simulink model "tractioncontrol_rmse22"  (R2022a)
settings: Solver=VariableStepAuto  StartTime=0.0  StopTime=48  RelTol=1e-3
values from neighbouring files (symbols this model uses):
  A = 1.08    [test_script.m]
  c = 0.008    [test_script.m]
  Cd = 1.02    [test_script.m]
  g = 9.81    [test_script.m]
  gr = 47/13    (= 3.61538461538)    [test_script.m]
  h_cg = .259    (= 0.259)    [test_script.m]
  h_d = h_cg    (= 0.259)    [test_script.m]
  J = 0.27    [test_script.m]
  m = 297    [test_script.m]
  r = 0.5588    [test_script.m]
  rho = 1.162    [test_script.m]
  wb = 1.53    [test_script.m]
undefined symbols (not defined in the file or in its folder): efficiency, front_wb, simulation_results, uff
libraries: slpidlib x2
settings Model: Creator=sahil  LastModifiedBy=sahil

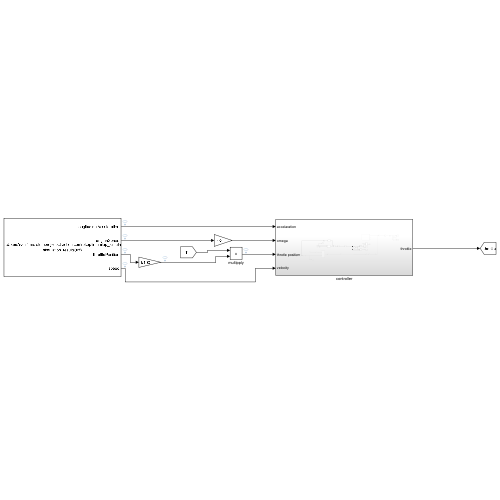
[thumbnail: Simulink's stored preview of the top-level diagram]
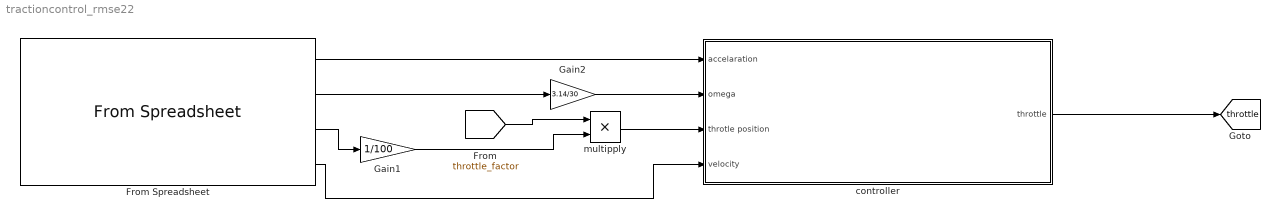
== system tractioncontrol_rmse22 ==
  From Spreadsheet : FromSpreadsheet  FileName=C:\Users\sahil\rms stuff\projects\traction control\optimumlap_simulations\simulation_results(uff).csv  SheetName=simulation_results(uff)
  Gain1 : Gain  Gain=1/100
  Gain2 : Gain  Gain=3.14/30
  controller : Subsystem
  multipply : Product  Inputs=**
  tag scope: throttle=global
  wires:
  From Spreadsheet/1 -> controller/1(accelaration)
  From Spreadsheet/3 -> Gain1/1
  controller/1(throttle) -> [throttle]
  From Spreadsheet/2 -> Gain2/1
  From Spreadsheet/4 -> controller/4(velocity)
  Gain2/1 -> controller/2(omega)
  [throttle_factor] -> multipply/1
  Gain1/1 -> multipply/2
  multipply/1 -> controller/3(throtle position)

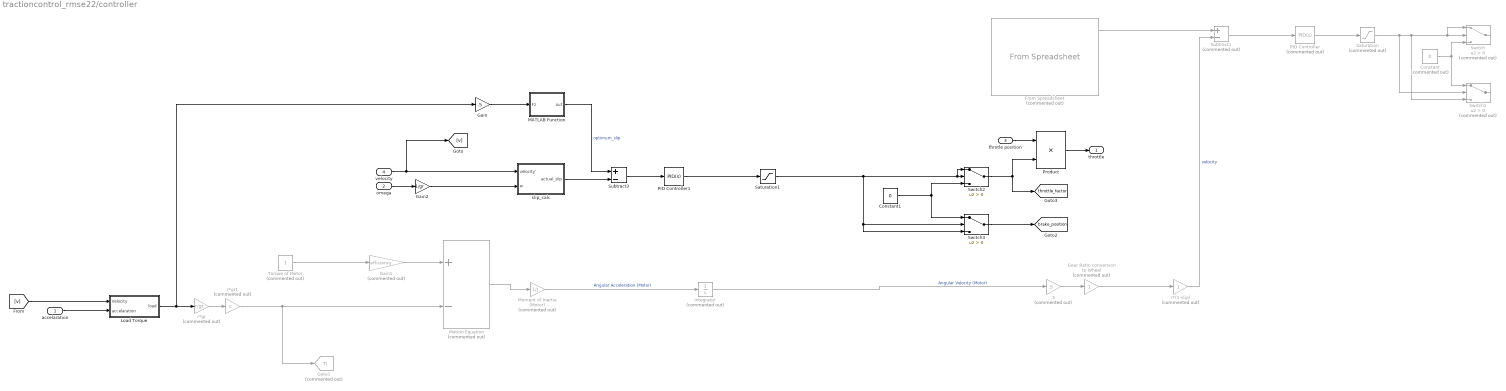
== system tractioncontrol_rmse22/controller ==
  accelaration : Inport
  omega : Inport  Port=2
  throtle position : Inport  Port=3
  velocity : Inport  Port=4
  .5 : Gain  Commented=on  Gain=.5
  Constant : Constant  Commented=on  Value=0
  Constant1 : Constant  Value=0
  From Spreadsheet : FromSpreadsheet  Commented=on  FileName=C:\Users\sahil\rms stuff\projects\traction control\optimumlap_simulations\simulation_resultsssss.csv  SheetName=simulation_resultsssss
  Gain : Gain  Gain=.5
  Gain1 : Gain  Commented=on  Gain=efficiency
  Gain2 : Gain  Gain=1/gr
  "Gear Ratio conversion to Wheel " : Gain  Commented=on
  Goto1 : Goto  Commented=on  GotoTag=Tl  TagVisibility=global
  Integrator : Integrator  Commented=on
  Load Torque : Subsystem
  MATLAB Function : MATLAB Function  TreatAsAtomicUnit=on
  Moment of Inertia (Motor) : Gain  Commented=on  Gain=1/J
  Motion Equation : Sum  Commented=on  Inputs=+-
  PID Controller : slpidlib/PID Controller  Commented=on  Controller=PID  Form=Parallel  TimeDomain=Continuous-time  UseExternalTs=off  SampleTime=-1  IntegratorMethod=Forward Euler  FilterMethod=Forward Euler  ControllerParametersSource=internal  P=1  I=1  UseKiTs=off  D=0  N=100  UseFilter=on  TunerSelectOption=Transfer Function Based (PID Tuner App)  InitialConditionSource=internal  InitialConditionForIntegrator=0  InitialConditionForFilter=0  DifferentiatorICPrevScaledInput=0  ExternalReset=none  TrackingMode=off  Kt=1  LimitOutput=off  SatLimitsSource=internal  UpperSaturationLimit=inf  LowerSaturationLimit=-inf  LinearizeAsGain=on  AntiWindupMode=none  Kb=1  POutMin=[]  POutMax=[]  IOutMin=[]  IOutMax=[]  DOutMin=[]  DOutMax=[]  NOutMin=[]  NOutMax=[]  SumOutMin=[]  SumOutMax=[]  SaturationOutMin=[]  SaturationOutMax=[]  PParamMin=[]  PParamMax=[]  IParamMin=[]  IParamMax=[]  DParamMin=[]  DParamMax=[]  NParamMin=[]  NParamMax=[]  KbParamMin=[]  KbParamMax=[]  KtParamMin=[]  KtParamMax=[]  KbOutMin=[]  KbOutMax=[]  KtOutMin=[]  KtOutMax=[]  IntegratorOutMin=[]  IntegratorOutMax=[]  FilterOutMin=[]  FilterOutMax=[]  SumI1OutMin=[]  SumI1OutMax=[]  SumI2OutMin=[]  SumI2OutMax=[]  SumI3OutMin=[]  SumI3OutMax=[]  SumI4OutMin=[]  SumI4OutMax=[]  SumDOutMin=[]  SumDOutMax=[]  DifferentiatorOutMin=[]  DifferentiatorOutMax=[]  FilterDiffOutCoefMin=[]  FilterDiffOutCoefMax=[]  ReciprocalOutMin=[]  ReciprocalOutMax=[]  SumDenOutMin=[]  SumDenOutMax=[]  SumNumOutMin=[]  SumNumOutMax=[]  DivideOutMin=[]  DivideOutMax=[]  UdiffTsProdOutMin=[]  UdiffTsProdOutMax=[]  NTsProdOutMin=[]  NTsProdOutMax=[]  UintegralTsProdOutMin=[]  UintegralTsProdOutMax=[]  UngainTsProdOutMin=[]  UngainTsProdOutMax=[]  IntegratorContinuousStateAttributes=''  IntegratorStateMustResolveToSignalObject=off  IntegratorRTWStateStorageClass=Auto  FilterContinuousStateAttributes=''  FilterStateMustResolveToSignalObject=off  FilterRTWStateStorageClass=Auto  ParallelPVariant=InternalParameters  IdealPVariant=Disabled  IVariant=InternalParameters  DVariant=InternalParameters  IntegratorVariant=Continuous  SatVariant=Disabled  AWVariant=Passthrough  PCopyVariant=Disabled  TRVariant=Disabled  FdbkBlocksVariant=Forward  IdealPFdbkVariant=Disabled  SatFdbkVariant=Disabled  DerivativeFilterVariant=ContFilter  NVariant=InternalParameters  NCopyVariant=Disabled  FilterICVariant=InternalICsFilter  IntegratorICVariant=InternalICs  ExternalResetVariant=Disabled  TRSumVariant=Passthrough  SumFdbkVariant=Disabled  SumVariant=Sum_PID  TsampFilterVariant=InternalTs  TsampNgainVariant=Passthrough  TsampIntegralVariant=Passthrough  ExternalSaturationOutDataTypeStr=Inherit: Same as second input  aMode=0
  PID Controller1 : slpidlib/PID Controller  Controller=PID  Form=Parallel  TimeDomain=Continuous-time  UseExternalTs=off  SampleTime=-1  IntegratorMethod=Forward Euler  FilterMethod=Forward Euler  ControllerParametersSource=internal  P=0.5  I=0.03  UseKiTs=off  D=0  N=100  UseFilter=on  TunerSelectOption=Transfer Function Based (PID Tuner App)  InitialConditionSource=internal  InitialConditionForIntegrator=0  InitialConditionForFilter=0  DifferentiatorICPrevScaledInput=0  ExternalReset=none  TrackingMode=off  Kt=1  LimitOutput=off  SatLimitsSource=internal  UpperSaturationLimit=inf  LowerSaturationLimit=-inf  LinearizeAsGain=on  AntiWindupMode=none  Kb=1  POutMin=[]  POutMax=[]  IOutMin=[]  IOutMax=[]  DOutMin=[]  DOutMax=[]  NOutMin=[]  NOutMax=[]  SumOutMin=[]  SumOutMax=[]  SaturationOutMin=[]  SaturationOutMax=[]  PParamMin=[]  PParamMax=[]  IParamMin=[]  IParamMax=[]  DParamMin=[]  DParamMax=[]  NParamMin=[]  NParamMax=[]  KbParamMin=[]  KbParamMax=[]  KtParamMin=[]  KtParamMax=[]  KbOutMin=[]  KbOutMax=[]  KtOutMin=[]  KtOutMax=[]  IntegratorOutMin=[]  IntegratorOutMax=[]  FilterOutMin=[]  FilterOutMax=[]  SumI1OutMin=[]  SumI1OutMax=[]  SumI2OutMin=[]  SumI2OutMax=[]  SumI3OutMin=[]  SumI3OutMax=[]  SumI4OutMin=[]  SumI4OutMax=[]  SumDOutMin=[]  SumDOutMax=[]  DifferentiatorOutMin=[]  DifferentiatorOutMax=[]  FilterDiffOutCoefMin=[]  FilterDiffOutCoefMax=[]  ReciprocalOutMin=[]  ReciprocalOutMax=[]  SumDenOutMin=[]  SumDenOutMax=[]  SumNumOutMin=[]  SumNumOutMax=[]  DivideOutMin=[]  DivideOutMax=[]  UdiffTsProdOutMin=[]  UdiffTsProdOutMax=[]  NTsProdOutMin=[]  NTsProdOutMax=[]  UintegralTsProdOutMin=[]  UintegralTsProdOutMax=[]  UngainTsProdOutMin=[]  UngainTsProdOutMax=[]  IntegratorContinuousStateAttributes=''  IntegratorStateMustResolveToSignalObject=off  IntegratorRTWStateStorageClass=Auto  FilterContinuousStateAttributes=''  FilterStateMustResolveToSignalObject=off  FilterRTWStateStorageClass=Auto  ParallelPVariant=InternalParameters  IdealPVariant=Disabled  IVariant=InternalParameters  DVariant=InternalParameters  IntegratorVariant=Continuous  SatVariant=Disabled  AWVariant=Passthrough  PCopyVariant=Disabled  TRVariant=Disabled  FdbkBlocksVariant=Forward  IdealPFdbkVariant=Disabled  SatFdbkVariant=Disabled  DerivativeFilterVariant=ContFilter  NVariant=InternalParameters  NCopyVariant=Disabled  FilterICVariant=InternalICsFilter  IntegratorICVariant=InternalICs  ExternalResetVariant=Disabled  TRSumVariant=Passthrough  SumFdbkVariant=Disabled  SumVariant=Sum_PID  TsampFilterVariant=InternalTs  TsampNgainVariant=Passthrough  TsampIntegralVariant=Passthrough  ExternalSaturationOutDataTypeStr=Inherit: Same as second input  aMode=0
  Product : Product
  Saturation : Saturate  Commented=on  UpperLimit=1  LowerLimit=-1
  Saturation1 : Saturate  UpperLimit=1  LowerLimit=-1
  Subtract1 : Sum  Commented=on  Inputs=+-
  Subtract3 : Sum  Inputs=+-
  Switch : Switch  Commented=on  Criteria=u2 > Threshold  SaturateOnIntegerOverflow=off  InputSameDT=off
  Switch1 : Switch  Commented=on  Criteria=u2 > Threshold  SaturateOnIntegerOverflow=off  InputSameDT=off
  Switch2 : Switch  Criteria=u2 > Threshold  SaturateOnIntegerOverflow=off  InputSameDT=off
  Switch3 : Switch  Criteria=u2 > Threshold  SaturateOnIntegerOverflow=off  InputSameDT=off
  Torque of Motor : Constant  Commented=on
  r*(1-slip) : Gain  Commented=on
  r*gr : Gain  Commented=on  Gain=r/gr
  r*gr1 : Gain  Commented=on  Gain=c
  slip_calc : Subsystem
  throttle : Outport
  tag scope: brake_position=global, throttle_factor=global
  wires:
  From Spreadsheet/1 -> Subtract1/1
  Product/1 -> throttle/1
  Torque of Motor/1 -> Gain1/1
  "Gear Ratio conversion to Wheel "/1 -> r*(1-slip)/1
  slip_calc/1(actual_slip) -> Subtract3/2
  Gain/1 -> MATLAB Function/1(Fz)
  r*(1-slip)/1 -> Subtract1/2  "velocity"
  throtle position/1 -> Product/1
  Motion Equation/1 -> Moment of Inertia (Motor)/1
  Moment of Inertia (Motor)/1 -> Integrator/1  "Angular Acceleration (Motor)"
  Integrator/1 -> .5/1  "Angular Velocity (Motor)"
  r*gr/1 -> r*gr1/1
  PID Controller/1 -> Saturation/1
  .5/1 -> "Gear Ratio conversion to Wheel "/1
  Gain1/1 -> Motion Equation/1
  Saturation/1 -> Switch1/2, Switch1/3, Switch/1, Switch/2
  Constant/1 -> Switch1/1, Switch/3
  MATLAB Function/1(out) -> Subtract3/1  "optimum_slip"
  PID Controller1/1 -> Saturation1/1
  Subtract3/1 -> PID Controller1/1
  Load Torque/1(load) -> Gain/1, r*gr/1
  Subtract1/1 -> PID Controller/1
  Saturation1/1 -> Switch3/2, Switch3/3, Switch2/1, Switch2/2
  omega/1 -> Gain2/1
  accelaration/1 -> Load Torque/2(accelaration)
  velocity/1 -> [v], slip_calc/1(velocity')
  [v] -> Load Torque/1(Velocity)
  Constant1/1 -> Switch2/3, Switch3/1
  Switch2/1 -> [throttle_factor], Product/2
  Switch3/1 -> [brake_position]
  r*gr1/1 -> Motion Equation/2, Goto1/1
  Gain2/1 -> slip_calc/2(w)

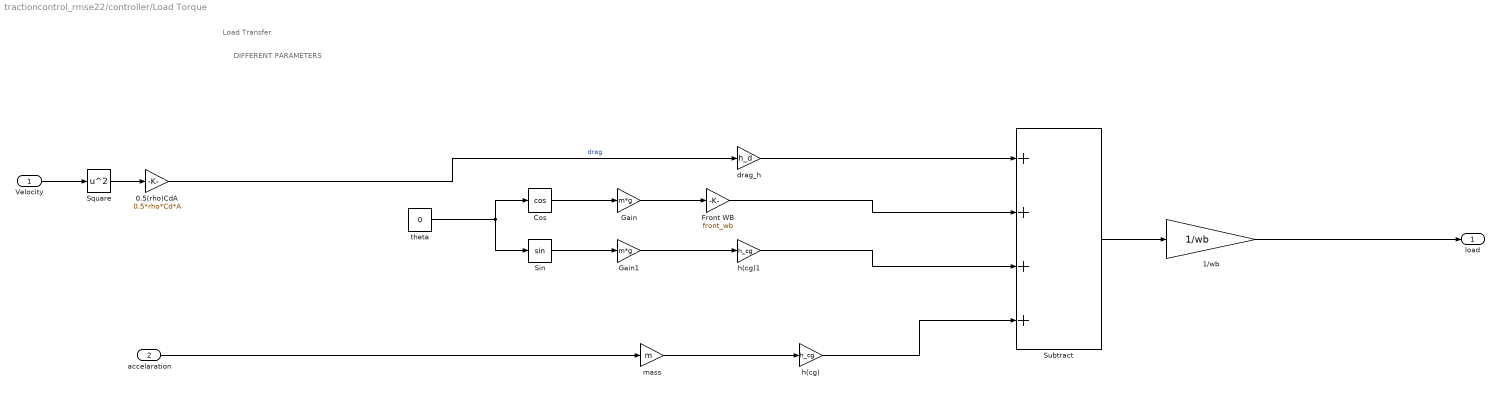
== system tractioncontrol_rmse22/controller/Load Torque ==
  note: Load Transfer
  note: DIFFERENT PARAMETERS
  Velocity : Inport
  accelaration : Inport  Port=2
  0.5(rho)CdA : Gain  Gain=0.5*rho*Cd*A
  1/wb : Gain  Gain=1/wb
  Cos : Trigonometry  Operator=cos
  Front WB : Gain  Gain=front_wb
  Gain : Gain  Gain=m*g
  Gain1 : Gain  Gain=m*g
  Sin : Trigonometry
  Square : Math  Operator=square
  Subtract : Sum  Inputs=++++
  drag_h : Gain  Gain=h_d
  h(cg) : Gain  Gain=h_cg
  h(cg)1 : Gain  Gain=h_cg
  mass : Gain  Gain=m
  theta : Constant  Value=0
  load : Outport
  wires:
  0.5(rho)CdA/1 -> drag_h/1  "drag"
  Velocity/1 -> Square/1
  1/wb/1 -> load/1
  Square/1 -> 0.5(rho)CdA/1
  Cos/1 -> Gain/1
  theta/1 -> Sin/1, Cos/1
  Sin/1 -> Gain1/1
  mass/1 -> h(cg)/1
  drag_h/1 -> Subtract/1
  Front WB/1 -> Subtract/2
  h(cg)1/1 -> Subtract/3
  h(cg)/1 -> Subtract/4
  Subtract/1 -> 1/wb/1
  accelaration/1 -> mass/1
  Gain/1 -> Front WB/1
  Gain1/1 -> h(cg)1/1

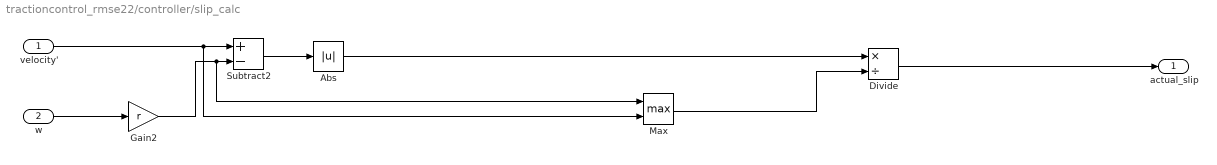
== system tractioncontrol_rmse22/controller/slip_calc ==
  velocity' : Inport
  w : Inport  Port=2
  Abs : Abs  SaturateOnIntegerOverflow=off
  Divide : Product  Inputs=*/
  Gain2 : Gain  Gain=r
  Max : MinMax  Function=max  Inputs=2
  Subtract2 : Sum  Inputs=+-
  actual_slip : Outport
  wires:
  Max/1 -> Divide/2
  velocity'/1 -> Max/2, Subtract2/1
  Gain2/1 -> Max/1, Subtract2/2
  w/1 -> Gain2/1
  Subtract2/1 -> Abs/1
  Abs/1 -> Divide/1
  Divide/1 -> actual_slip/1

== matlab function tractioncontrol_rmse22/controller/MATLAB Function ==
  data: Fz input; out output
function out=packeja(Fz)
    
    a1=-2.13*(10^-5);
    a2=1.144;
    a3=4.96*(10^-5);
    a4=.226;
    a5=6.9*(10^-5);
    a6=-6*(10^-9);
    a7=5.6*(10*(-5));
    a8=.486;
    
    lambda=0:.005:1;
    Cx=1.65;
    Dx=a1*Fz*Fz+a2*Fz;
    func1=(a3*Fz*Fz+a4*Fz)*exp(-a5*Fz);
    Bx=func1/(Cx*Dx);
    Ex=a6*Fz*Fz+a7*Fz+a8;
    G=Bx*lambda;
    func2=G*(1-Ex)+Ex*atan(G);
    Fx=Dx*sin(Cx*atan(func2));
    plot(lambda,Fx)
    [~,I]=max(Fx);
    slip=lambda(I);
    out=slip;

end
